simulink library "StateCtrlLib"  (R2018b)
settings: Solver=VariableStepAuto  StartTime=0.0  StopTime=10.0  RelTol=1e-3
settings Model: Creator=sn2xws  LastModifiedBy=sn2xws

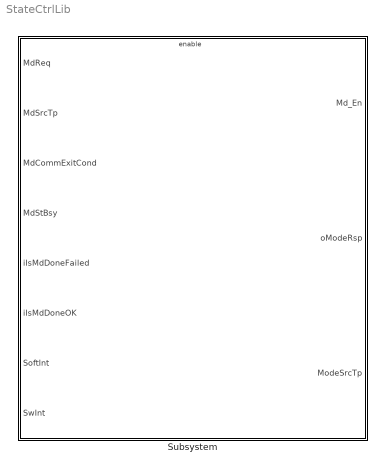
== system StateCtrlLib ==
  Subsystem : Subsystem

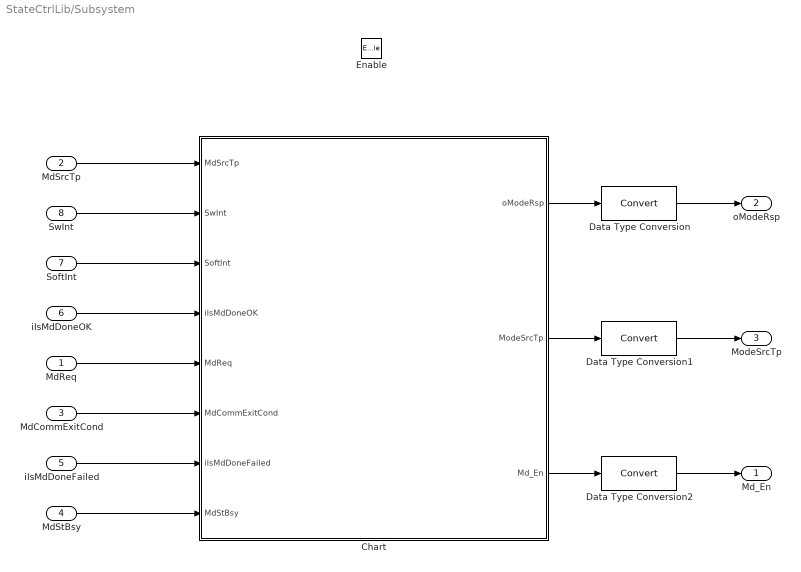
== system StateCtrlLib/Subsystem ==
  MdReq : Inport
  MdSrcTp : Inport  Port=2
  MdCommExitCond : Inport  Port=3
  MdStBsy : Inport  Port=4
  iIsMdDoneFailed : Inport  Port=5
  iIsMdDoneOK : Inport  Port=6
  SoftInt : Inport  Port=7
  SwInt : Inport  Port=8
  Enable : EnablePort  StatesWhenEnabling=reset
  Chart : Stateflow chart  TreatAsAtomicUnit=on
  Data Type Conversion : DataTypeConversion
  Data Type Conversion1 : DataTypeConversion
  Data Type Conversion2 : DataTypeConversion
  Md_En : Outport
  oModeRsp : Outport  Port=2
  ModeSrcTp : Outport  Port=3
  wires:
  Chart/3(Md_En) -> Data Type Conversion2/1
  iIsMdDoneFailed/1 -> Chart/7(iIsMdDoneFailed)
  MdCommExitCond/1 -> Chart/6(MdCommExitCond)
  SoftInt/1 -> Chart/3(SoftInt)
  MdReq/1 -> Chart/5(MdReq)
  iIsMdDoneOK/1 -> Chart/4(iIsMdDoneOK)
  MdStBsy/1 -> Chart/8(MdStBsy)
  MdSrcTp/1 -> Chart/1(MdSrcTp)
  SwInt/1 -> Chart/2(SwInt)
  Chart/1(oModeRsp) -> Data Type Conversion/1
  Chart/2(ModeSrcTp) -> Data Type Conversion1/1
  Data Type Conversion/1 -> oModeRsp/1
  Data Type Conversion1/1 -> ModeSrcTp/1
  Data Type Conversion2/1 -> Md_En/1

== stateflow chart StateCtrlLib/Subsystem/Chart ==
  settings: executeAtInitialization=1
  state MdOngoing
    en:Md_En = 1;
    en:ModeSrcTp = MdSrcTp;
    en:oModeRsp = MdRspLocal1.MdRsp_RecallOngoing;
  state MdIlde
    en:Md_En =0;
    en:ModeSrcTp =SrcReqTp1.SrcReqTp_None;
  (default) -> MdIlde
  MdIlde -> MdOngoing : [(MdReq)&&MdStBsy ==0]
  MdOngoing -> MdIlde [order 1] : [hasChangedTo(SoftInt,true)]{oModeRsp = MdRspLocal1.MdRsp_RecallUnsuccessfully_LocalInterrupt;}
  MdOngoing -> MdIlde [order 2] : [hasChangedTo(SwInt,true)]{oModeRsp =MdRspLocal1.MdRsp_RecallUnsuccessfully_LocalInterrupt; }
  MdOngoing -> MdIlde [order 3] : [hasChangedTo(iIsMdDoneOK,true)]{oModeRsp =MdRspLocal1.MdRsp_RecallSuccessfully;}
  MdOngoing -> MdIlde [order 4] : [MdCommExitCond]{oModeRsp = MdRspLocal1.MdRsp_RecallUnsuccessfully_Error;}
  MdOngoing -> MdIlde [order 5] : [hasChangedTo(iIsMdDoneFailed,true)]{oModeRsp = MdRspLocal1.MdRsp_RecallUnsuccessfully_Error;}
  data: MdSrcTp input; SwInt input; SoftInt input; iIsMdDoneOK input; MdReq input; MdCommExitCond input; iIsMdDoneFailed input; MdStBsy input; oModeRsp output Enum: MdRspLocal1; ModeSrcTp output Enum: SrcReqTp1; Md_En output boolean
